simulink model "SoC_ColumbCounting_Ex2"  (R2024b)
settings: Solver=ode3  StartTime=0.0  StopTime=3600  RelTol=1e-3
undefined symbols (not defined in the file): Ion, Lithium
libraries: spsBatteryLib x16, spsSeriesRLCBranchLib x3, spsCurrentMeasurementLib x1, spsGroundLib x1, spsSeriesRLCLoadLib x1, spsVoltageMeasurementLib x1, sps_lib x1
settings Model: Creator=balaj  LastModifiedBy=balaj
settings SolverCC: ZeroCrossControl=DisableAll

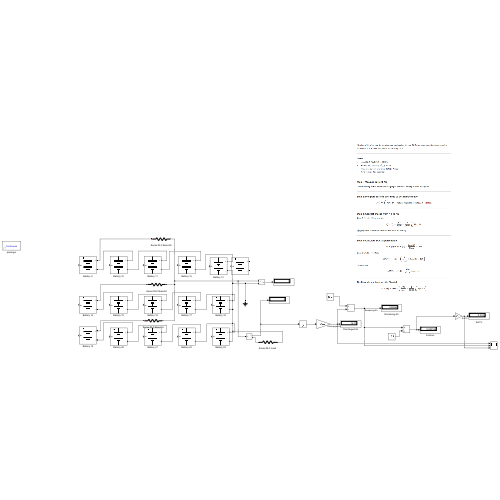
[thumbnail: Simulink's stored preview of the top-level diagram]
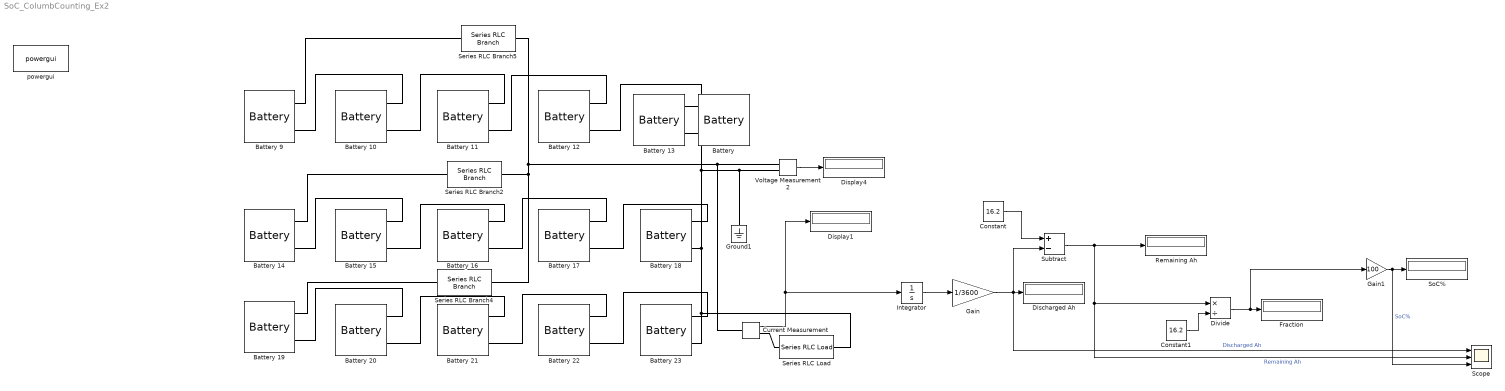
== system SoC_ColumbCounting_Ex2 ==
  Battery : spsBatteryLib/Battery  BatType=Lithium-Ion  NomV=7.2  NomQ=5.4  SOC=100  Batt_Tr=30  PresetModel=on  MaxQ=5.4  MinV=5.4  FullV=8.3807  Dis_rate=2.3478  R=0.013333  Normal_OP=4.8835  expZone="[7.7788      0.2653]"
  Battery {9..23} (15 alike) : spsBatteryLib/Battery  BatType=Lithium-Ion  NomV=3.2  NomQ=5.4  SOC=100  Batt_Tr=30  PresetModel=off  MaxQ=5.4  MinV=2.4  FullV=3.7  Dis_rate=2.3478  R=0.0059259  Normal_OP=4.8835  expZone="[3.4572      0.2653]"
  Constant : Constant  Value=16.2
  Constant1 : Constant  Value=16.2
  Current Measurement : spsCurrentMeasurementLib/Current Measurement  PhasorSimulation=off  OutputType=Complex  PSBequivalent=0
  Discharged Ah : Display
  Display1 : Display
  Display4 : Display
  Divide : Product  Inputs=*/
  Fraction : Display
  Gain : Gain  Gain=1/3600
  Gain1 : Gain  Gain=100
  Ground1 : spsGroundLib/Ground  LConnTagsString=a
  Integrator : Integrator
  Remaining Ah : Display
  Scope : Scope  NumInputPorts=3
  Series RLC Branch2 : spsSeriesRLCBranchLib/Series RLC Branch  LConnTagsString=__new0  RConnTagsString=__new0  BranchType=R  Resistance=0.01  Inductance=1e-3  SetiL0=off  InitialCurrent=0  Capacitance=1e-6  Setx0=off  InitialVoltage=0  Measurements=None
  Series RLC Branch4 : spsSeriesRLCBranchLib/Series RLC Branch  LConnTagsString=__new0  RConnTagsString=__new0  BranchType=R  Resistance=0.01  Inductance=1e-3  SetiL0=off  InitialCurrent=0  Capacitance=1e-6  Setx0=off  InitialVoltage=0  Measurements=None
  Series RLC Branch5 : spsSeriesRLCBranchLib/Series RLC Branch  LConnTagsString=__new0  RConnTagsString=__new0  BranchType=R  Resistance=0.01  Inductance=1e-3  SetiL0=off  InitialCurrent=0  Capacitance=1e-6  Setx0=off  InitialVoltage=0  Measurements=None
  "Series RLC Load " : spsSeriesRLCLoadLib/Series RLC Load  LConnTagsString=a  RConnTagsString=__new0  NominalVoltage=18.5  NominalFrequency=50  ActivePower=500  InductivePower=0  CapacitivePower=0  Setx0=off  InitialVoltage=0  SetiL0=off  InitialCurrent=0  Measurements=None  LoadType=constant Z
  SoC% : Display
  Subtract : Sum  Inputs=+-
  Voltage Measurement2 : spsVoltageMeasurementLib/Voltage Measurement  PhasorSimulation=off  OutputType=Complex  PSBequivalent=0
  powergui : sps_lib/powergui  Priority=1  SimulationMode=Continuous  SampleTime=50e-6  frequency=60  Iterations=50  frequencyindice=0  Pbase=100e6  ErrMax=1e-4  UnitsV=kV  UnitsW=MW  buscounter=0  FunctionMessages=off  echomessages=off  EnableUseOfTLC=off  CurrentSourceSwitches=off  DisableSnubberDevices=off  DisableRonSwitches=off  DisableVfSwitches=off  DisplayEquations=off  AutomaticDiscreteSolvers=off  SolverType=Tustin/Backward Euler (TBE)  Interpol=off  ExternalGateDelay=off  methode=off  Ts=100  x0status=blocks  SPID=on  SwTol=0  HookPort=off  NonlinearTolerance=1e-4  nMaxIteration=100  ContinueOnMaxIteration=off  RestoreLinks=warning  ResistiveCurrentMeasurement=off  Frange=[0:2:500]  Ylog=off  Xlog=on  ShowGrid=off  save=off  variable=ZData  structure=0  ZoomFFT=off  StartTime=0.0  cycles=1  DisplayStyle=1  fundamental=60  FreqAxis=off  MaxFrequency=1000  frequencyindicesteady=1  RmsSteady=1  display=off
  wires:
  Voltage Measurement2/1 -> Display4/1
  Current Measurement/1 -> Display1/1, Integrator/1
  Integrator/1 -> Gain/1
  Gain/1 -> Scope/1, Subtract/2, Discharged Ah/1  "Discharged Ah"
  Constant/1 -> Subtract/1
  Subtract/1 -> Scope/2, Divide/1, Remaining Ah/1  "Remaining Ah"
  Constant1/1 -> Divide/2
  Divide/1 -> Gain1/1, Fraction/1
  Gain1/1 -> Scope/3, SoC%/1  "SoC%"
  connections:
  Battery 10/LConn1 -- Battery 9/LConn2
  Battery 11/LConn1 -- Battery 10/LConn2
  Battery 12/LConn1 -- Battery 11/LConn2
  Battery 12/LConn2 -- Battery 13/LConn1
  Battery 15/LConn1 -- Battery 14/LConn2
  Battery 15/LConn2 -- Battery 16/LConn1
  Battery 17/LConn1 -- Battery 16/LConn2
  Battery 17/LConn2 -- Battery 18/LConn1
  Battery 20/LConn1 -- Battery 19/LConn2
  Battery 21/LConn1 -- Battery 20/LConn2
  Battery 21/LConn2 -- Battery 22/LConn1
  Battery 22/LConn2 -- Battery 23/LConn1
  Series RLC Branch5/LConn1 -- Battery 9/LConn1
  Series RLC Branch2/LConn1 -- Battery 14/LConn1
  Series RLC Branch4/LConn1 -- Battery 19/LConn1
  Series RLC Branch5/RConn1 -- Current Measurement/LConn1 -- Voltage Measurement2/LConn1 -- Series RLC Branch4/RConn1 -- Series RLC Branch2/RConn1
  Battery 13/LConn2 -- Voltage Measurement2/LConn2 -- Ground1/LConn1 -- "Series RLC Load "/RConn1 -- Battery 23/LConn2 -- Battery 18/LConn2
  Current Measurement/RConn1 -- "Series RLC Load "/LConn1
